simulink model "VehiclePlant"  (R2022b)
settings: Solver=VariableStepAuto  StartTime=0.0  StopTime=10.0  RelTol=1e-3
values from neighbouring files (symbols this model uses):
  L = 2.8    [main.m]
  Vx = V_interval{i}(2)    [main.m]
settings Model: Creator=mirko  LastModifiedBy=ludovicaperroni
settings SolverCC: AlgebraicLoopSolver=TrustRegion
settings OptimizationCC: ReuseModelBlockBuffer=on
settings DebuggingCC: UnconnectedInputMsg=warning  UnconnectedOutputMsg=warning  UnconnectedLineMsg=warning
settings ModelReferenceCC: EnableRefExpFcnMdlSchedulingChecks=on
settings SFSimCC: CustomCodeUndefinedFunction=UseInterfaceOnly

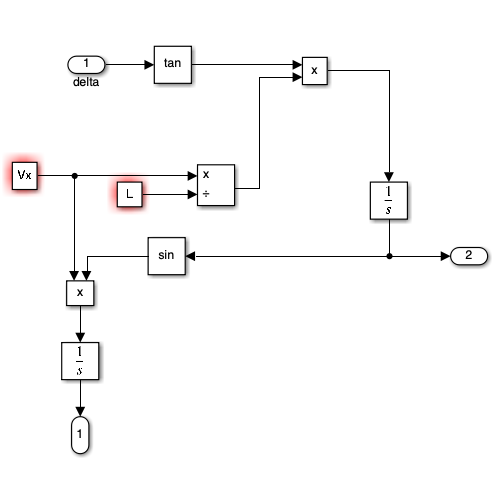
[thumbnail: Simulink's stored preview of the top-level diagram]
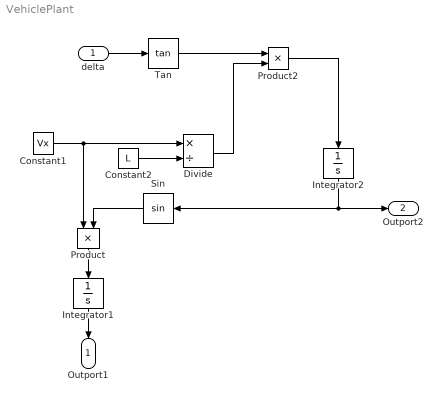
== system VehiclePlant ==
  delta : Inport
  Constant1 : Constant  Value=Vx
  Constant2 : Constant  Value=L
  Divide : Product  Inputs=*/
  Integrator1 : Integrator
  Integrator2 : Integrator
  Product : Product
  Product2 : Product
  Sin : Trigonometry
  Tan : Trigonometry  Operator=tan
  Outport1 : Outport  VectorParamsAs1DForOutWhenUnconnected=off
  Outport2 : Outport  Port=2  VectorParamsAs1DForOutWhenUnconnected=off
  wires:
  Constant2/1 -> Divide/2
  Tan/1 -> Product2/1
  Sin/1 -> Product/2
  Integrator2/1 -> Sin/1, Outport2/1
  Product/1 -> Integrator1/1
  Product2/1 -> Integrator2/1
  Constant1/1 -> Product/1, Divide/1
  Divide/1 -> Product2/2
  delta/1 -> Tan/1
  Integrator1/1 -> Outport1/1
